simulink model "template_poloha"  (Simulink 7.0)
settings: Solver=ode3  StartTime=0.0  StopTime=Tsim  FixedStep=Tvz  RelTol=1e-3
values from neighbouring files (symbols this model uses):
  Ki = 0.825    [mojeMerani02.mat]    (also in mojeMerani03.mat = 0.5; mojeMerani04.mat = 0.45; mojeMerani05.mat = 0.3; mojeMerani06i.mat = 0.3836)
  Kp = 4    [mojeMerani02.mat]    (also in mojeMerani03.mat = 6; mojeMerani04.mat; mojeMerani05.mat = 3.5; mojeMerani06i.mat = 1.7885)
  Kv = 0.1226    [mojeMerani02.mat]    (also in mojeMerani03.mat; mojeMerani04.mat; mojeMerani05.mat = 0.1; mojeMerani06i.mat = 0.0611)
  Mmax = 5    [mojeMerani02.mat]    (also in mojeMerani03.mat; mojeMerani04.mat; mojeMerani05.mat; mojeMerani06i.mat)
  Mn = 6.48    [mojeMerani02.mat]    (also in mojeMerani03.mat; mojeMerani04.mat; mojeMerani05.mat; mojeMerani06i.mat)
  poloha1 = 3.14159265359    [mojeMerani02.mat]    (also in mojeMerani03.mat; mojeMerani04.mat; mojeMerani05.mat; mojeMerani06i.mat)
  poloha2 = 6.28318530718    [mojeMerani02.mat]    (also in mojeMerani03.mat; mojeMerani04.mat; mojeMerani05.mat; mojeMerani06i.mat)
  Tsim = 5    [mojeMerani02.mat]    (also in mojeMerani03.mat; mojeMerani04.mat; mojeMerani05.mat; mojeMerani06i.mat)
  Tvz = 0.004    [mojeMerani02.mat]    (also in mojeMerani03.mat; mojeMerani04.mat; mojeMerani05.mat; mojeMerani06i.mat)
undefined symbols (not defined in the file or in its folder): DiscIntNeverNeededParam, Humusoft, MF624
libraries: rtwinlib x3, simulink x2
settings Model: Creator=Student  LastModifiedBy=STU_ABB  SimulationMode=external  ExtModeTrigDuration=6000
settings DebuggingCC: SaveWithParameterizedLinksMsg=none  SignalResolutionControl=TryResolveAllWithWarning  MultiTaskDSMMsg=warning  MultiTaskCondExecSysMsg=none
settings RTWCC: SystemTargetFile=rtwin.tlc  TemplateMakefile=rtwin.tmf  Description=Real-Time Windows Target  ProcessScript=rtwin_make_rtw_hook  IncludeERTFirstTime=on
settings RTWinTargetCC: TargetFcnLib=ansi_tfl_tmw.mat  GenFloatMathFcnCalls=ANSI_C  ModelReferenceCompliant=off  CompOptLevelCompliant=off  PortableWordSizes=off  CCOptimize=on

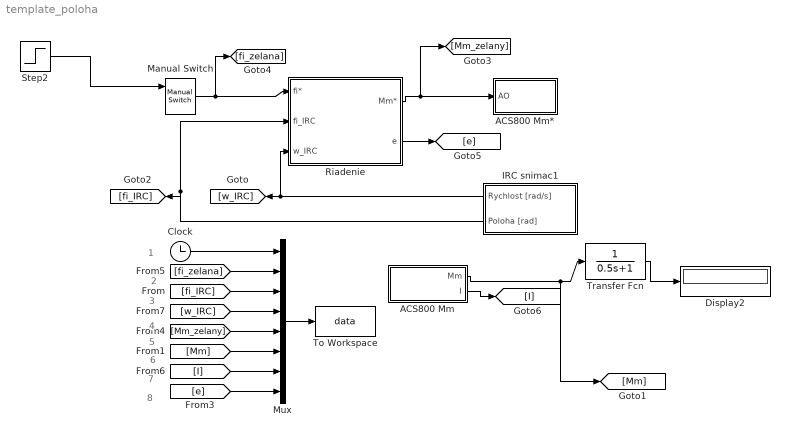
== system template_poloha ==
  note: 1
  note: 2
  note: 3
  note: 4
  note: 5
  note: 6
  note: 7
  note: 8
  ACS800 Mm : Subsystem  mask{AI=0, Posun=-0.012, Zosilnenie=Mn/10, Tvz=Tvz}
      mask prompts: AI "Cislo analogoveho vstupu na karte"; Posun "Offset vstupu"; Zosilnenie "Zosilenie vstupu"; Tvz "Perioda vzorkovania"
  ACS800 Mm* : Subsystem  mask{AO=1, Prevod=10/Mn, Tvz=Tvz, Tsim=Tsim}
      mask prompts: AO "Cislo analogoveho vystupu na karte"; Prevod "Zosilnenie Vystupu"; Tvz "Perioda vzorkovania"; Tsim "Doba simulacie"
  Clock : Clock
      settings: Decimation=10
  Display2 : Display
  IRC snimac1 : Subsystem  Orientation=left  mask{NIRC=2500, Tvz=Tvz}
      mask prompts: NIRC "Pocet impulzov IRC na otacku"; Tvz "Perioda vzorkovania"
  Manual Switch : simulink/Signal Routing/Manual Switch  SystemSampleTime=-1  sw=1  action=0  varsize=off
  Mux : Mux  Inputs=8
  Riadenie : Subsystem  TreatAsAtomicUnit=on
  Step2 : Step  Before=poloha1  After=poloha2  SampleTime=Tvz
  To Workspace : ToWorkspace  VariableName=data  SampleTime=Tvz  SaveFormat=Array
  Transfer Fcn : TransferFcn  Denominator=[0.5 1]
  wires:
  Manual Switch/1 -> [fi_zelana], Riadenie/1(fi*)
  Riadenie/1(Mm*) -> [Mm_zelany], ACS800 Mm*/1(AO)
  Riadenie/2(e) -> [e]
  ACS800 Mm/1(Mm) -> Transfer Fcn/1, [Mm]
  Transfer Fcn/1 -> Display2/1
  Step2/1 -> Manual Switch/1
  IRC snimac1/2(Poloha [rad]) -> Riadenie/2(fi_IRC), [fi_IRC]
  IRC snimac1/1(Rychlost [rad/s]) -> Riadenie/3(w_IRC), [w_IRC]
  Clock/1 -> Mux/1
  [fi_zelana] -> Mux/2
  [fi_IRC] -> Mux/3
  Mux/1 -> To Workspace/1
  [w_IRC] -> Mux/4
  [Mm_zelany] -> Mux/5
  [Mm] -> Mux/6
  [I] -> Mux/7
  [e] -> Mux/8
  ACS800 Mm/2(I) -> [I]

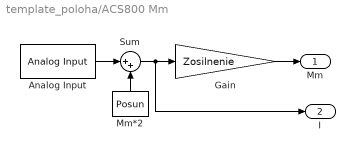
== system template_poloha/ACS800 Mm ==
  Analog Input : rtwinlib/Analog Input  SampleTime=Tvz  DrvName=Humusoft/MF624  DrvAddress=4294967295  DrvOptions=0  Channels=1  RangeMode=1  VoltRange=1  DataType=1
      settings: AttributesFormatString=Humusoft\nMF624 [auto]
  Gain : Gain  Gain=Zosilnenie  ParameterDataType=sfix(16)  ParameterScaling=2^0  OutDataType=sfix(16)  OutScaling=2^0  SampleTime=Tvz
  Mm*2 : Constant  Orientation=up  Value=Posun  OutDataType=sfix(16)  OutScaling=2^0  SampleTime=Tvz
  Sum : Sum  Inputs=|++  OutDataType=sfix(16)  OutScaling=2^0
  Mm : Outport
  I : Outport  Port=2
  wires:
  Gain/1 -> Mm/1
  Mm*2/1 -> Sum/2
  Sum/1 -> Gain/1, I/1
  Analog Input/1 -> Sum/1

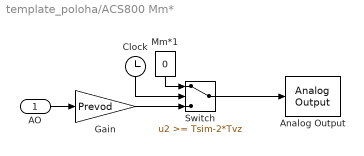
== system template_poloha/ACS800 Mm* ==
  AO : Inport
  Analog Output : rtwinlib/Analog Output  SampleTime=Tvz  DrvName=Humusoft/MF624  DrvAddress=4294967295  DrvOptions=0  Channels=AO  RangeMode=1  VoltRange=1  InitialValue=0  FinalValue=[]
      settings: AttributesFormatString=Humusoft\nMF624 [auto]
  Clock : Clock
      settings: Orientation=down
  Gain : Gain  Gain=Prevod  ParameterDataType=sfix(16)  ParameterScaling=2^0  OutDataType=sfix(16)  OutScaling=2^0  SampleTime=Tvz
  Mm*1 : Constant  Orientation=down  Value=0  OutDataType=sfix(16)  OutScaling=2^0  SampleTime=Tvz
  Switch : Switch  Threshold=Tsim-2*Tvz  OutDataType=sfix(16)  OutScaling=2^0  SampleTime=Tvz
  wires:
  Gain/1 -> Switch/3
  AO/1 -> Gain/1
  Mm*1/1 -> Switch/1
  Clock/1 -> Switch/2
  Switch/1 -> Analog Output/1

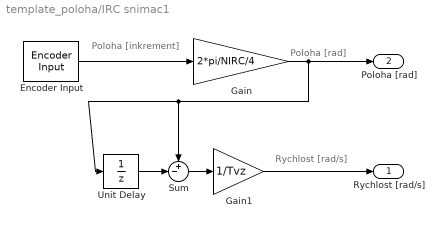
== system template_poloha/IRC snimac1 ==
  note: Rychlost [rad/s]
  note: Poloha [rad]
  note: Poloha [inkrement]
  Encoder Input : rtwinlib/Encoder Input  SampleTime=Tvz  DrvName=Humusoft/MF624  DrvAddress=4294967295  DrvOptions=0  Channels=2  QuadMode=3  IndexPulse=2  InputFilter=Inf  DataType=1
      settings: AttributesFormatString=Humusoft\nMF624 [auto]
  Gain : Gain  Gain=2*pi/NIRC/4  ParameterDataType=sfix(16)  ParameterScaling=2^0  OutDataType=sfix(16)  OutScaling=2^0
  Gain1 : Gain  Gain=1/Tvz  ParameterDataType=sfix(16)  ParameterScaling=2^0  OutDataType=sfix(16)  OutScaling=2^0  SampleTime=Tvz
  Sum : Sum  Inputs=+-|  OutDataType=sfix(16)  OutScaling=2^0  SampleTime=Tvz
  Unit Delay : UnitDelay  SampleTime=Tvz
  Rychlost [rad/s] : Outport
  Poloha [rad] : Outport  Port=2
  wires:
  Gain1/1 -> Rychlost [rad/s]/1
  Sum/1 -> Gain1/1
  Unit Delay/1 -> Sum/2
  Gain/1 -> Sum/1, Unit Delay/1, Poloha [rad]/1
  Encoder Input/1 -> Gain/1

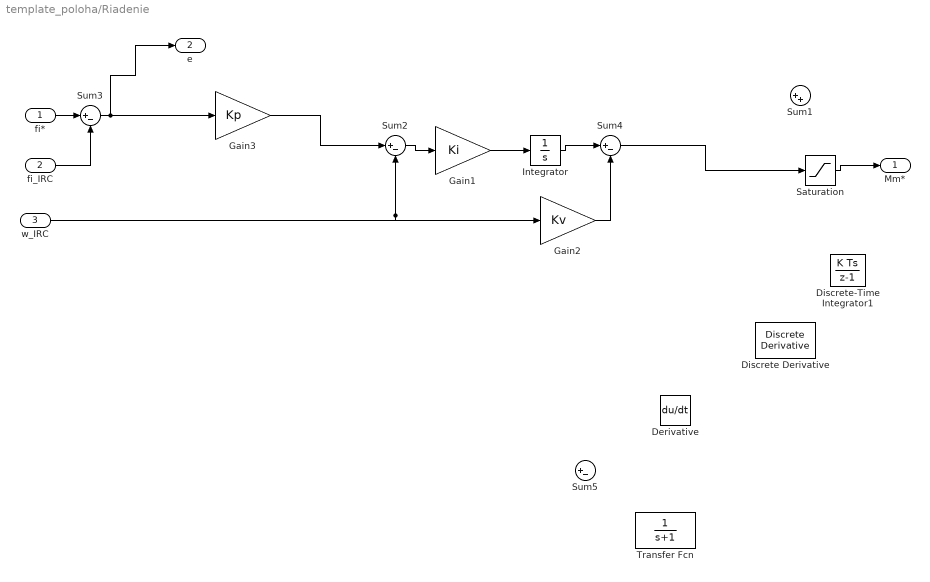
== system template_poloha/Riadenie ==
  fi* : Inport  OutDataType=sfix(16)  OutScaling=2^0
  fi_IRC : Inport  Port=2  OutDataType=sfix(16)  OutScaling=2^0
  w_IRC : Inport  Port=3  OutDataType=sfix(16)  OutScaling=2^0
  Derivative : Derivative
  Discrete Derivative : simulink/Discrete/Discrete Derivative  SystemSampleTime=-1  gainval=1.0  ICPrevScaledInput=0.0  OutMin=[]  OutMax=[]  OutDataType=sfix(16)  OutScaling=2^-10  DoSatur=off
  Discrete-Time Integrator1 : DiscreteIntegrator  gainval=1  SampleTime=Tvz  OutDataType=fixdt(1, 16)  OutScaling=2^0  ICPrevOutput=DiscIntNeverNeededParam  ICPrevScaledInput=DiscIntNeverNeededParam
  Gain1 : Gain  Gain=Ki  ParameterDataType=fixdt(1, 16)  ParameterScaling=2^0  OutDataType=fixdt(1, 16)  OutScaling=2^0
  Gain2 : Gain  Gain=Kv  ParameterDataType=fixdt(1, 16)  ParameterScaling=2^0  OutDataType=fixdt(1, 16)  OutScaling=2^0
  Gain3 : Gain  Gain=Kp  ParameterDataType=fixdt(1, 16)  ParameterScaling=2^0  OutDataType=fixdt(1, 16)  OutScaling=2^0
  Integrator : Integrator
  Saturation : Saturate  UpperLimit=Mmax  LowerLimit=-Mmax  OutDataType=fixdt(1, 16)  OutScaling=2^0
  Sum1 : Sum  Inputs=|++  OutDataType=sfix(16)  OutScaling=2^0
  Sum{2..5} (4 alike) : Sum  Inputs=|+-  OutDataType=sfix(16)  OutScaling=2^0
  Transfer Fcn : TransferFcn  Denominator=[1 1]
  Mm* : Outport  OutDataType=sfix(16)  OutScaling=2^0
  e : Outport  Port=2  OutDataType=sfix(16)  OutScaling=2^0
  wires:
  Saturation/1 -> Mm*/1
  fi*/1 -> Sum3/1
  Sum3/1 -> Gain3/1, e/1
  fi_IRC/1 -> Sum3/2
  Gain3/1 -> Sum2/1
  w_IRC/1 -> Sum2/2, Gain2/1
  Sum2/1 -> Gain1/1
  Gain1/1 -> Integrator/1
  Integrator/1 -> Sum4/1
  Gain2/1 -> Sum4/2
  Sum4/1 -> Saturation/1
